simulink model "VTOLAutopilotController"  (R2025a)
settings: configuration reference "VTOLConfiguration" (kept outside this file)
undefined symbols (not defined in the file): Back_Transition_Rate, const, control, controlParams, ControlSampleTime, CriticalTiltAngle, DiscIntNeverNeededParam, dspblkCoreblockFVToolHelper, Fading_time, flightState, FSState, FWControlParams, FWTrimSpeed, gcbh, HoverMission, ReferenceFilterDen, ReferenceFilterNum, tilt_max, tiltIni, TransitioncontrolGains, uavParam, uavParams, VTOLcontrolGains, w_trim, WindDownRate
libraries: simulink x43, slpidlib x35, uavalgslib x7, simulink_extras x1
(part 8 of 8)

== system VTOLAutopilotController/Guidance Test Bench/ControlType/Guidance Testbench/Guidance Logic/Guidance Stateflow/Guidance Mode Selector/GuidanceLogic.WP/Dist2WP/Subsystem ==
  V : Inport
  Dot Product1 : DotProduct  OutDataTypeStr=Inherit: Inherit via internal rule
  Product : Product  Inputs=*/
  Saturation : Saturate  UpperLimit=inf  LowerLimit=0.00001
  Sqrt : Sqrt
  V_unit : Outport
  wires:
  V/1 -> Dot Product1/2, Dot Product1/1, Product/1
  Sqrt/1 -> Product/2
  Dot Product1/1 -> Saturation/1
  Saturation/1 -> Sqrt/1
  Product/1 -> V_unit/1

== matlab function VTOLAutopilotController/Guidance Test Bench/ControlType/Guidance Testbench/Guidance Logic/Guidance Stateflow/Guidance Mode Selector/GuidanceLogic.Land.ToLand/MATLAB Function ==
  data: FromWP input Bus: doubleUavPathManager size=1; wps output; ToWP input Bus: doubleUavPathManager size=1
function wps = getLandingWaypoint(FromWP, ToWP)

persistent outWPS

if isempty(outWPS)
    outWPS = double(zeros(2,4));
end

outWPS(1,:) = [FromWP.position' FromWP.params(4)];
outWPS(2,:) = [ToWP.position(1:2)' FromWP.position(3) ToWP.params(4)];

wps = outWPS;

== matlab function VTOLAutopilotController/Guidance Test Bench/ControlType/Guidance Testbench/Guidance Logic/Guidance Stateflow/Guidance Mode Selector/GuidanceLogic.Land.Descend/MATLAB Function ==
  data: FromWP input Bus: doubleUavPathManager size=1; wps output; ToWPPos input size=[3 1]; ToWPParam input size=[4 1]
function wps = getLandingWaypoint(FromWP, ToWPPos, ToWPParam)

persistent outWPS

if isempty(outWPS)
    outWPS = double(zeros(2,4));
end

outWPS(1,:) = [FromWP.position' FromWP.params(4)];
outWPS(2,:) = [reshape(ToWPPos,1,[]), ToWPParam(4)];

wps = outWPS;

== matlab function VTOLAutopilotController/Low level controller/Fixed Wing Controller/Fixed Wing Controller Module/Fixed Wing Controller Simulation/Attitude Controller/Pitch Roll Controller/Turn Coordinator/MATLAB Function ==
  data: rollSP input; rSP output; pitchSP input; airSpeed input
function rSP = fcn(rollSP, pitchSP, airSpeed)
    yawRateSP = tan(rollSP)*9.81/max(airSpeed,5);
    rSP = yawRateSP*cos(pitchSP)*cos(rollSP);
end

== matlab function VTOLAutopilotController/Low level controller/Fixed Wing Controller/Fixed Wing Controller Module/Fixed Wing Controller Simulation/Lateral Guidance Logic/MATLAB Function ==
  data: courseSP input; lacc output; course input; rollSP output; groundSpeed input; L1 input
function [lacc, rollSP] = fcn(courseSP, course, groundSpeed, L1)
eta = courseSP - course;

% wrap -pi to pi
eta = mod(eta, 2*pi);
if eta>pi
    eta = eta - 2*pi;
end

% cap eta to -pi/2 to pi/2
eta = min(eta, pi/2);
eta = max(eta, -pi/2);

lacc = 2*(groundSpeed^2)/L1*sin(eta);

rollSP = atan(lacc/9.81);

== matlab function VTOLAutopilotController/Low level controller/Fixed Wing Controller/Fixed Wing Controller Module/Fixed Wing Controller Tuning/Subsystem2/MATLAB Function ==
  data: phi input; y output; theta input
function y = fcn(phi,theta)

y=zeros(3,3);
y=[1 sin(phi)*tan(theta) cos(phi)*tan(theta); 0 cos(phi) -sin(phi); 0 sin(phi)/cos(theta) cos(phi)/cos(theta)];
end

== matlab function VTOLAutopilotController/Low level controller/Fixed Wing Controller/Fixed Wing Controller Module/Fixed Wing Controller Tuning/Lateral Guidance Logic/MATLAB Function ==
  data: courseSP input; lacc output; course input; rollSP output; groundSpeed input; L1 input
function [lacc, rollSP] = fcn(courseSP, course, groundSpeed, L1)
eta = courseSP - course;

% wrap -pi to pi
eta = mod(eta, 2*pi);
if eta>pi
    eta = eta - 2*pi;
end

% cap eta to -pi/2 to pi/2
eta = min(eta, pi/2);
eta = max(eta, -pi/2);

lacc = 2*(groundSpeed^2)/L1*sin(eta);

rollSP = atan(lacc/9.81);

== matlab function VTOLAutopilotController/Low level controller/Fixed Wing Controller/Fixed Wing Controller Module/Fixed Wing Controller Tuning/Attitude Controller/Pitch Roll Controller/Turn Coordinator/MATLAB Function ==
  data: rollSP input; rSP output; pitchSP input; airSpeed input
function rSP = fcn(rollSP, pitchSP, airSpeed)
    yawRateSP = tan(rollSP)*9.81/max(airSpeed,5);
    rSP = yawRateSP*cos(pitchSP)*cos(rollSP);
end

== matlab function VTOLAutopilotController/Guidance Test Bench/ControlType/Guidance Testbench/Guidance Logic/Guidance Stateflow/Guidance Mode Selector/GuidanceLogic.BackTransition.BackTransition/MATLAB Function ==
  data: Vb input; tilt input; flag output
function flag = fcn(Vb,tilt)
tiltConditionMet=abs(tilt)<1e-1;
velocityConditionMet=abs(norm([Vb(1) 0 0]))<15;

flag=tiltConditionMet&velocityConditionMet;
end

== stateflow chart VTOLAutopilotController/Guidance Test Bench/ControlType/Guidance Testbench/Guidance Logic/Guidance Stateflow/Guidance Mode Selector ==
  settings: updateMethod=DISCRETE  sampleTime=4*controlParams.ControlSampleTime
  state GuidanceLogic
    state FixedWingEntry
      state FixedWingStabilize
        %.. stabilize fixed-wing transition once done
        en:
        FlightMode=flightState.FixedWing;
        ControlMode.attitude = 1;
        ControlMode.airspeedaltitude = 0;
        ControlMode.lateralguidance = 0;
        ControlMode.transitioncondition = uint8(0);
        state Stabilize
      state FixedWingFlight
        %.. enable fixed-wing outer loop
        en:
        ControlMode.airspeedaltitude = 1;
        ControlMode.attitude = 1;
        ControlMode.lateralguidance = 1;
        state GuidanceInitialization
      (default) -> FixedWingStabilize
      FixedWingStabilize -> FixedWingFlight : after(3,sec)
    state FIXED_WING_WAYPOINT
      en:
      ControlMode.airspeedaltitude = 1;
      ControlMode.attitude = 1;
      ControlMode.lateralguidance = 1;
      state WAYPOINT
    state Start
      %.. initialize guidance mode selector
      en:
      %.. set flight mode to hover
      FlightMode = PresetMode;
      %.. set default settings
      %.. control mode
      ControlMode.airspeedaltitude = 0;
      ControlMode.attitude = 0;
      ControlMode.lateralguidance = 0;
      ControlMode.transitioncondition = 0;
      %.. setpoint initialization
      HoverSP.localposition = [0; 0; 0];
      HoverSP.yaw = 0;
      VTOLSP.roll = 0;
      VTOLSP.pitch = 0;
      VTOLSP.yaw = 0;
      FixedWingSP.roll = 0;
      FixedWingSP.pitch = 0;
      FixedWingSP.yaw = 0;
      FixedWingSP.airspeed = 30.867;
      FixedWingSP.flap = 0;
      AACSP.airspeed = 30.867;
      AACSP.L1 = 300;
      AACSP.altitude = 0;
      AACSP.course = 0;
      AACSP.climbrate = 0;
    state FIXED_WING_ORBIT
      en:
      ControlMode.airspeedaltitude = 1;
      ControlMode.attitude = 1;
      ControlMode.lateralguidance = 1;
      state ORBIT
    state HOVER_ENTRY
      en:
      FlightMode=flightState.Hover;
      ControlMode.intransition=1;
    state Takeoff
    state WP
    state Orbit
    state PreTransition
      en:
      FlightMode=flightState.BackTransition;
      ControlMode.lateralguidance = 1;
      ControlMode.attitude = 1;
      ControlMode.airspeedaltitude = 1;
      % Setpoint init
      AACSP.L1 = 400;
      AACSP.airspeed = 0;
      AACSP.altitude = altitudeHold;
      AACSP.course = courseHold;
      state StabilizeFixedWingBack
    state BackTransition
      HoverSP.localposition = [States.Xe(1); States.Xe(2); altitudeHold];
      HoverSP.yaw = 0;
      state BackTransition
    state ForwardTransitionComplete
      %.. complete forward transition and switch to fixed-wing mode
      Status = uint8(1);
      ControlMode.transitioncondition = uint8(1);
    state ForwardTransitionBegin
    state ForwardTransitionIntermediate
    state Land
      state Descend
      state ToLand
      (default) -> ToLand
      ToLand -> Descend : [(norm(Pose(1:2)-ToWP.position(1:2)) <= 3)]
    (default) -> Start
    FixedWingFlight -> ORBIT [order 1] : [(mode==3)]
        | {Status= uint8(0);}
    Start -> (junction 5)
    FixedWingFlight -> WAYPOINT [order 2] : [(mode==2)]
        | {Status=uint8(0);}
    (junction 5) -> FIXED_WING_ORBIT [order 6] : [(mode==3)&&(FlightMode==flightState.FixedWing)]
        | {Status=uint8(0);}
    (junction 255) -> HOVER_ENTRY
    (junction 5) -> (junction 255) [order 4] : [(FlightMode==flightState.BackTransition)]
    (junction 262) -> FixedWingEntry
    (junction 5) -> (junction 262) [order 3] : [(FlightMode==flightState.Transition)]
        | {ControlMode.intransition=0;
        | ControlMode.transitioncondition = uint8(0);}
    HOVER_ENTRY -> (junction 12) : [after(2,sec)]{ControlMode.intransition=0;}
    (junction 257) -> FIXED_WING_WAYPOINT
    Takeoff -> WP : [Pose(3) <= ToWP.position(3)+10.0]
        | {Status = uint8(1);}
    GuidanceLogic -> (junction 5) : [(hasChanged(mode))]
    (junction 5) -> Takeoff [order 5] : [(mode == 1)&&(FlightMode==flightState.Hover)]
        | {ControlMode.intransition=0;}
    (junction 5) -> (junction 257) [order 2] : [(mode==2)&&(FlightMode==flightState.FixedWing)]
        | {Status=uint8(0);}
    (junction 5) -> (junction 260) [order 1] : [(mode==6)&&(FlightMode==flightState.FixedWing)]
        | {courseHold = States.course;
        | altitudeHold = -States.Xe(3);}
    (junction 5) -> (junction 12) [order 7] : [FlightMode==flightState.Hover]
        | {ControlMode.intransition=0;}
    (junction 12) -> WP [order 1] : [(mode==2)]
    (junction 12) -> (junction 17) [order 2]
    (junction 260) -> PreTransition
    (junction 17) -> Orbit [order 1] : [(mode==3)]
    (junction 17) -> (junction 22) [order 2]
    PreTransition -> GuidanceLogic.BackTransition : [after(10,sec)]
        | {FlightMode=flightState.BackTransition;
        | ControlMode.intransition=1; }
    ForwardTransitionIntermediate -> ForwardTransitionComplete : [FWDTransitionCompleteMet(States,VFWDTransition2)]
    ForwardTransitionBegin -> ForwardTransitionIntermediate : [FWDTransitionConditionMet(States,VFWDTransition1)]
        | {ControlMode.attitude = 1;
        | ControlMode.airspeedaltitude = 0;
        | ControlMode.lateralguidance = 0;}
    (junction 22) -> ForwardTransitionBegin [order 1] : [(mode==6)&&(FlightMode==flightState.Hover)]
        | {FlightMode=flightState.Transition;
        | ControlMode.intransition=1;
        | ControlMode.transitioncondition=uint8(0);}
    (junction 22) -> Land [order 2] : [(mode==4)]
  (default) -> GuidanceLogic
  data: sf_internal_action_state_placeholder_data local double size=1 =0; sf_internal_action_state_placeholder_data local double size=1 =0; sf_internal_action_state_placeholder_data local double size=1 =0; sf_internal_action_state_placeholder_data local double size=1 =0; sf_internal_action_state_placeholder_data local double size=1 =0; sf_internal_action_state_placeholder_data local double size=1 =0; sf_internal_action_state_placeholder_data local double size=1 =0; sf_internal_action_state_placeholder_data local double size=1 =0; sf_internal_action_state_placeholder_data local double size=1 =0; sf_internal_action_state_placeholder_data local double size=1 =0; sf_internal_action_state_placeholder_data local double size=1 =0; sf_internal_action_state_placeholder_data local double size=1 =0; sf_internal_action_state_placeholder_data local double size=1 =0; TransitionSt function_input Bus: GuidanceStates; valid function_output; Vtransition function_input; TransitionSt function_input Bus: GuidanceStates; valid function_output; Vtransition function_input; TransitionSt function_input Bus: GuidanceStates; valid function_output; Vtransition function_input; GuidanceMode output Enum: GdncModeType; mode input; ToWP input Bus: doubleUavPathManager; Status output uint8; FromWP input Bus: doubleUavPathManager; Pose input; States input; AACSP output Bus: AAC; FixedWingSP output Bus: FixedWingCommandBus; ControlMode output Bus: ControlMode; FlightMode output; PresetMode input; courseHold local; altitudeHold local; HoverSP output Bus: LAPY; zGround parameter; Ground input; VFWDTransition1 input double; VFWDTransition2 input; VTOLSP output Bus: VTOLCommandBus; ModeFDBK input
  function valid=FWDTransitionCompleteMet(TransitionSt,Vtransition):
    | function valid=FWDTransitionCompleteMet(TransitionSt,Vtransition)
    | %wingsLevel
    | if(TransitionSt.Tilt>=1.57)&&(vecnorm(TransitionSt.Ve)>Vtransition)
    |    valid=true;
    | else
    |     valid=false;
    | end
    | end
  function valid=FWDTransitionConditionMet(TransitionSt,Vtransition):
    | function valid=FWDTransitionConditionMet(TransitionSt,Vtransition)
    | %wingsLevel
    | if(vecnorm(TransitionSt.Ve)>Vtransition)
    |    valid=true;
    | else
    |     valid=false;
    | end
    | end
  function valid=BWDTransitionConditionMet(TransitionSt,Vtransition):
    | function valid=BWDTransitionConditionMet(TransitionSt,Vtransition)
    | %wingsLevel
    | if(vecnorm(TransitionSt.Ve)<Vtransition)
    |    valid=true;
    | else
    |     valid=false;
    | end
    | end

== matlab function VTOLAutopilotController/Guidance Test Bench/ControlType/Guidance Testbench/Guidance Logic/Guidance Stateflow/Guidance Mode Selector/GuidanceLogic.WP/MATLAB Function ==
  data: FromWP input Bus: doubleUavPathManager size=1; wps output; ToWP input Bus: doubleUavPathManager size=1
function wps = getWaypointMission(FromWP, ToWP)

persistent outWPS

if isempty(outWPS)
    outWPS = double(zeros(2,4));
end

outWPS(1,:) = [FromWP.position' FromWP.params(1)];
outWPS(2,:) = [ToWP.position' ToWP.params(1)];

wps = outWPS;

== matlab function VTOLAutopilotController/Guidance Test Bench/ControlType/Guidance Testbench/Guidance Logic/Guidance Stateflow/Guidance Mode Selector/GuidanceLogic.FIXED_WING_WAYPOINT.WAYPOINT/MATLAB Function ==
  data: toWP input; wps output; fromWP input; alt output
function [wps, alt]= fcn(toWP, fromWP)
    wps = zeros(2,3); %#ok<PREALL> 
    wps = [fromWP'; toWP'];
    alt = -toWP(3);
end

== matlab function VTOLAutopilotController/Low level controller/Fixed Wing Controller/Fixed Wing Controller Module/Fixed Wing Controller Simulation/Subsystem2/MATLAB Function ==
  data: phi input; y output; theta input
function y = fcn(phi,theta)

y=zeros(3,3);
y=[1 sin(phi)*tan(theta) cos(phi)*tan(theta); 0 cos(phi) -sin(phi); 0 sin(phi)/cos(theta) cos(phi)/cos(theta)];
end

== stateflow chart VTOLAutopilotController/Guidance Test Bench/ControlType/Manual Control/Command Interface/Basic Control  Switching ==
  state STATE_MACHINE
    state DEFAULT
      en:
      controlMode.lateralGuidance=1;
      controlMode.airspeedAltitude=1;
      controlMode.attitude=1;
      controlMode.manual=0;
      controlMode.armed=0;
      controlMode.inTransition=0;
    state TRANSITION
      controlMode.lateralGuidance=1;
      controlMode.airspeedAltitude=1;
      controlMode.attitude=1;
      controlMode.manual=0;
      controlMode.armed=0;
      controlMode.inTransition=1;
      controlMode.TransitionCondition=0;
    (default) -> DEFAULT
    STATE_MACHINE -> DEFAULT [order 2] : [hasChanged(FlightMode)]
    STATE_MACHINE -> TRANSITION [order 1] : [hasChanged(FlightMode)&&((FlightMode==flightState.Transition)||(FlightMode==flightState.BackTransition))]
    TRANSITION -> STATE_MACHINE [order 2] : [backConditioMet(States)&&(FlightMode==flightState.BackTransition)]
        | {controlMode.TransitionCondition=1;
        | controlMode.inTransition=0;}
    TRANSITION -> STATE_MACHINE [order 1] : [transitionConditionMet(States,Vt)&&(FlightMode==flightState.Transition)]
        | {controlMode.TransitionCondition=1;
        | controlMode.inTransition=0;}
  data: TransitionStates function_input Bus: GuidanceStates; valid function_output; Vtransition function_input; TransitionStates function_input Bus: GuidanceStates; valid function_output; controlMode output Bus: controlMode; FlightMode input; States input; Vt parameter double
  function valid=transitionConditionMet(TransitionStates,Vtransition):
    | function valid=transitionConditionMet(TransitionStates,Vtransition)
    | %wingsLevel
    | if((States.Tilt>=1.57)&&(vecnorm(States.Ve)>Vt))
    |    valid=true;
    | else
    |     valid=false;
    | end
    | end
  function valid=backConditioMet(TransitionStates):
    | function valid=backConditioMet(TransitionStates)
    | %wingsLevel
    | if(vecnorm(States.Ve)<1e-1)
    |    valid=true;
    | else
    |     valid=false;
    | end
    | end
